simulink model "SingleAgentQUAV"  (R2018b)
settings: Solver=ode1  StartTime=0.0  StopTime=10  FixedStep=tstep  RelTol=1e-3
InitFcn:
  | initSim;
StopFcn:
  | plotSimSolution;
undefined symbols (not defined in the file or in its folder): m, problem, tstep
settings Model: Creator=yn15  LastModifiedBy=dan
settings OptimizationCC: LifeSpan=inf
settings DebuggingCC: SFUnexpectedBacktrackingDiag=warning  SFNoUnconditionalDefaultTransitionDiag=warning  SFExecutionAtInitializationDiag=none
settings SFSimCC: SimUseLocalCustomCode=off
settings RTWCC: RTWUseLocalCustomCode=off
settings CodeAppCC: StateflowObjectComments=on
settings GRTTargetCC: TargetLangStandard=C89/C90 (ANSI)
settings ConfigComp: CovMetricSettings=dw  CovHtmlReporting=on  CovSaveCumulativeToWorkspaceVar=on  CovSaveSingleToWorkspaceVar=on  CovExternalEMLEnable=off

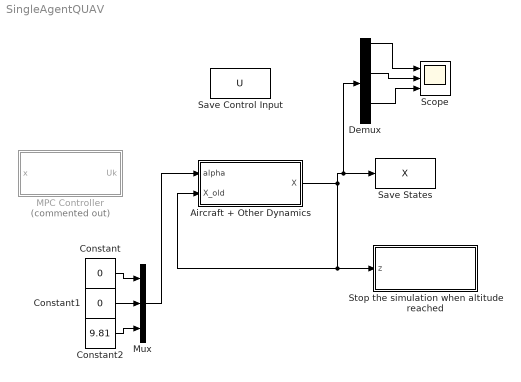
== system SingleAgentQUAV ==
  Aircraft + Other Dynamics : Subsystem
  Constant : Constant  Value=0
  Constant1 : Constant  Value=0
  Constant2 : Constant  Value=9.81
  Demux : Demux  Outputs=6
  "MPC Controller " : Subsystem  Commented=on
  Mux : Mux  Inputs=3
  Save Control Input : ToWorkspace  VariableName=U  SampleTime=-1
      settings: Save2DSignal=2-D array (concatenate along first dimension)
  Save States : ToWorkspace  VariableName=X  SampleTime=-1
  Scope : Scope  NumInputPorts=3
  "Stop the simulation when altitude reached " : Subsystem
  wires:
  Aircraft + Other Dynamics/1(X) -> Demux/1, Save States/1, "Stop the simulation when altitude reached "/1(z), Aircraft + Other Dynamics/2("X_old ")
  Constant/1 -> Mux/1
  Constant1/1 -> Mux/2
  Constant2/1 -> Mux/3
  Mux/1 -> Aircraft + Other Dynamics/1(alpha)
  Demux/1 -> Scope/1
  Demux/3 -> Scope/2
  Demux/5 -> Scope/3

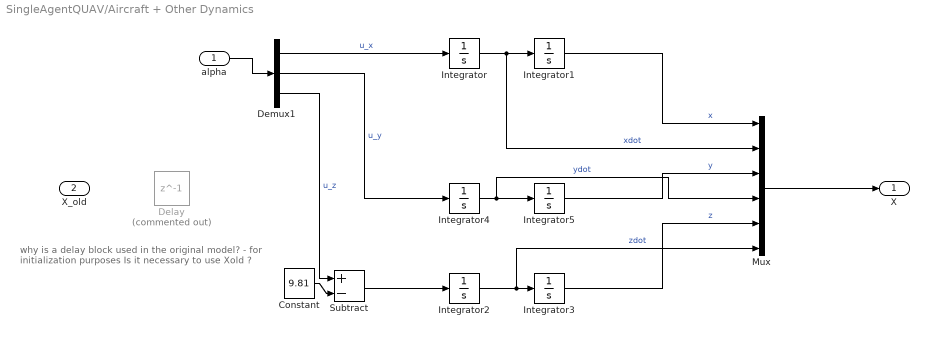
== system SingleAgentQUAV/Aircraft + Other Dynamics ==
  note: why is a delay block used in the original model?
      | - for initialization purposes
      |
      | Is it necessary to use Xold ?
  alpha : Inport
  "X_old " : Inport  Port=2
  Constant : Constant  Value=9.81
  Delay : Delay  Commented=on  DelayLength=1  InitialCondition=[problem.states.x0]
  Demux1 : Demux  Outputs=3
  Integrator{,1..2,4..5} (5 alike) : Integrator
  Integrator3 : Integrator  InitialCondition=5
  Mux : Mux  Inputs=6
  Subtract : Sum  Inputs=+-
  X : Outport
  wires:
  alpha/1 -> Demux1/1
  Mux/1 -> X/1
  Constant/1 -> Subtract/2
  Integrator/1 -> Mux/2, Integrator1/1  "xdot"
  Integrator2/1 -> Mux/6, Integrator3/1  "zdot"
  Integrator4/1 -> Mux/4, Integrator5/1  "ydot"
  Demux1/1 -> Integrator/1  "u_x"
  Integrator1/1 -> Mux/1  "x"
  Demux1/2 -> Integrator4/1  "u_y"
  Integrator5/1 -> Mux/3  "y"
  Demux1/3 -> Subtract/1  "u_z"
  Subtract/1 -> Integrator2/1
  Integrator3/1 -> Mux/5  "z"

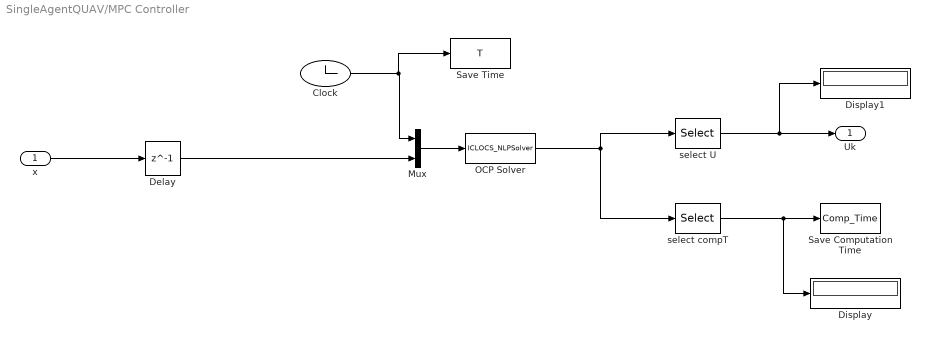
== system SingleAgentQUAV/MPC Controller  ==
  x : Inport
  Clock : Clock
  Delay : Delay  DelayLength=1  InitialCondition=[problem.states.x0]
  Display : Display
  Display1 : Display
  Mux : Mux  Inputs=2
  OCP Solver : MATLABFcn  MATLABFcn=ICLOCS_NLPSolver  OutputDimensions=m+2
  "Save Computation Time " : ToWorkspace  VariableName=Comp_Time  SampleTime=tstep
      settings: Save2DSignal=2-D array (concatenate along first dimension)
  Save Time : ToWorkspace  VariableName=T  SampleTime=-1
      settings: Save2DSignal=2-D array (concatenate along first dimension)
  select U : Selector  IndexOptions=Index vector (dialog)  Indices=3:m+2  OutputSizes=1
  select compT : Selector  IndexOptions=Index vector (dialog)  Indices=2  OutputSizes=1
  Uk : Outport
  wires:
  select U/1 -> Display1/1, Uk/1
  x/1 -> Delay/1
  OCP Solver/1 -> select compT/1, select U/1
  Clock/1 -> Save Time/1, Mux/1
  Mux/1 -> OCP Solver/1
  Delay/1 -> Mux/2
  select compT/1 -> Display/1, "Save Computation Time "/1

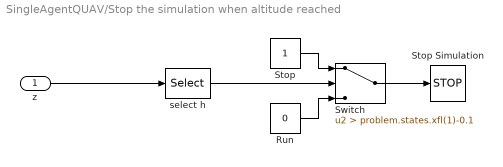
== system SingleAgentQUAV/Stop the simulation when altitude reached  ==
  z : Inport
  Run : Constant  Value=0
  Stop : Constant
  Stop Simulation : Stop
  Switch : Switch  Criteria=u2 > Threshold  Threshold=problem.states.xfl(1)-0.1
  select h : Selector  IndexOptions=Index vector (dialog)  Indices=1  OutputSizes=1
  wires:
  Switch/1 -> Stop Simulation/1
  z/1 -> select h/1
  Stop/1 -> Switch/1
  Run/1 -> Switch/3
  select h/1 -> Switch/2
